simulink model "untitled"  (R2022b)
settings: Solver=VariableStepAuto  StartTime=0.0  StopTime=10.0  RelTol=1e-3
undefined symbols (not defined in the file): Ion, Lithium, Ts, Ts_Power
libraries: spsSeriesRLCBranchLib x7, spsMeanLib x5, spsFirstOrderFilterLib x4, spsStairGeneratorLib x4, spsDiodeLib x4, spsPWMGeneratorDCDCLib x3, spsBoostConverterLib x2, spsPVArrayLib x2, spsIGBTLib x2, spsPowerPositiveSequenceLib x1, spsRMSLib x1, spsBatteryLib x1
settings Model: Creator=刘明炜  LastModifiedBy=刘明炜

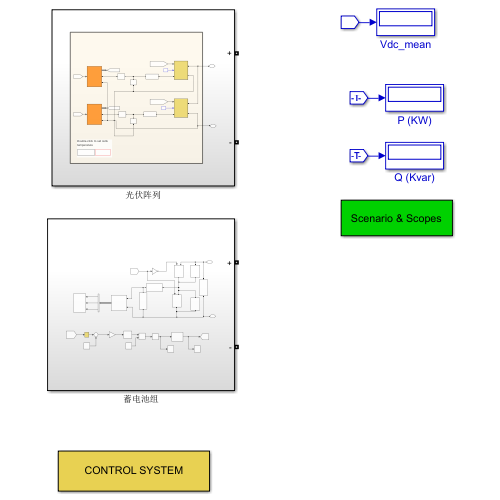
[thumbnail: Simulink's stored preview of the top-level diagram]
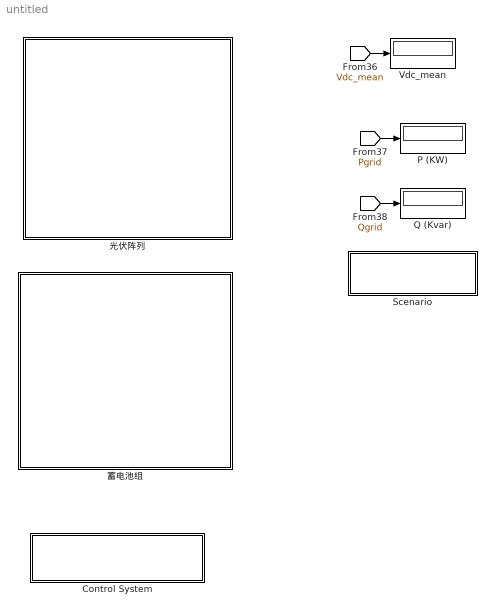
== system untitled ==
  Control System : Subsystem
      mask Display: disp('CONTROL SYSTEM')
  P (KW) : Display
      settings: Format=bank  Decimation=200
  Q (Kvar) : Display
      settings: Format=bank  Decimation=200
  Scenario : Subsystem
      mask Display: disp('Scenario & Scopes')
  Vdc_mean : Display
      settings: Decimation=200
  光伏阵列 : Subsystem
  蓄电池组 : Subsystem
  wires:
  [Pgrid] -> P (KW)/1
  [Vdc_mean] -> Vdc_mean/1
  [Qgrid] -> Q (Kvar)/1

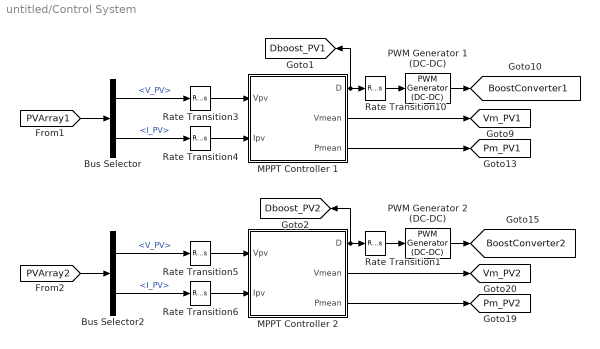
== system untitled/Control System ==
  Bus Selector : BusSelector  OutputSignals=V_PV,I_PV
  Bus Selector2 : BusSelector  OutputSignals=V_PV,I_PV
  MPPT Controller 1 : Subsystem  mask(MPPT Controller - Perturb and Observe algorithm (PandO)){Dinit=0.35, Dlimits=[0.8, 0.3], deltaD=60e-6, Fc=1000, Ts=Ts}
      mask prompts: Dinit "Duty cycle (D) initial value"; Dlimits "D limits [Upper, Lower]"; deltaD "Increment value for PandO algorithm"; Fc "Measurement filter cutoff frequency (Hz)"; Ts "Sample time (s)"
      mask init:
      | Dmax=Dlimits(1);
      | Dmin=Dlimits(2);
  MPPT Controller 2 : Subsystem  mask(MPPT Controller - Perturb and Observe algorithm (PandO)){Dinit=0.55, Dlimits=[0.8, 0.47], deltaD=60e-6, Fc=1000, Ts=Ts}
      mask prompts: Dinit "Duty cycle (D) initial value"; Dlimits "D limits [Upper, Lower]"; deltaD "Increment value for PandO algorithm"; Fc "Measurement filter cutoff frequency (Hz)"; Ts "Sample time (s)"
      mask init:
      | Dmax=Dlimits(1);
      | Dmin=Dlimits(2);
  PWM Generator 1 (DC-DC) : spsPWMGeneratorDCDCLib/PWM Generator (DC-DC)  Fsw=5000  Ts=Ts_Power
  PWM Generator 2 (DC-DC) : spsPWMGeneratorDCDCLib/PWM Generator (DC-DC)  Fsw=5000  Ts=Ts_Power
  Rate Transition1 : RateTransition  OutPortSampleTime=Ts_Power
  Rate Transition10 : RateTransition  OutPortSampleTime=Ts_Power
  Rate Transition{3..6} (4 alike) : RateTransition  OutPortSampleTime=Ts
  tag scope: BoostConverter1=global, BoostConverter2=global, Dboost_PV1=global, Dboost_PV2=global, Pm_PV1=global, Pm_PV2=global, Vm_PV1=global, Vm_PV2=global
  wires:
  MPPT Controller 2/2(Vmean) -> [Vm_PV2]
  Bus Selector2/1 -> Rate Transition5/1  "<V_PV>"
  Rate Transition3/1 -> MPPT Controller 1/1(Vpv)
  Rate Transition4/1 -> MPPT Controller 1/2(Ipv)
  Bus Selector/2 -> Rate Transition4/1  "<I_PV>"
  MPPT Controller 2/3(Pmean) -> [Pm_PV2]
  MPPT Controller 1/1(D) -> [Dboost_PV1], Rate Transition10/1
  Bus Selector/1 -> Rate Transition3/1  "<V_PV>"
  Bus Selector2/2 -> Rate Transition6/1  "<I_PV>"
  Rate Transition1/1 -> PWM Generator 2 (DC-DC)/1
  Rate Transition6/1 -> MPPT Controller 2/2(Ipv)
  MPPT Controller 1/3(Pmean) -> [Pm_PV1]
  MPPT Controller 1/2(Vmean) -> [Vm_PV1]
  Rate Transition10/1 -> PWM Generator 1 (DC-DC)/1
  MPPT Controller 2/1(D) -> [Dboost_PV2], Rate Transition1/1
  Rate Transition5/1 -> MPPT Controller 2/1(Vpv)
  PWM Generator 1 (DC-DC)/1 -> [BoostConverter1]
  PWM Generator 2 (DC-DC)/1 -> [BoostConverter2]
  [PVArray1] -> Bus Selector/1
  [PVArray2] -> Bus Selector2/1

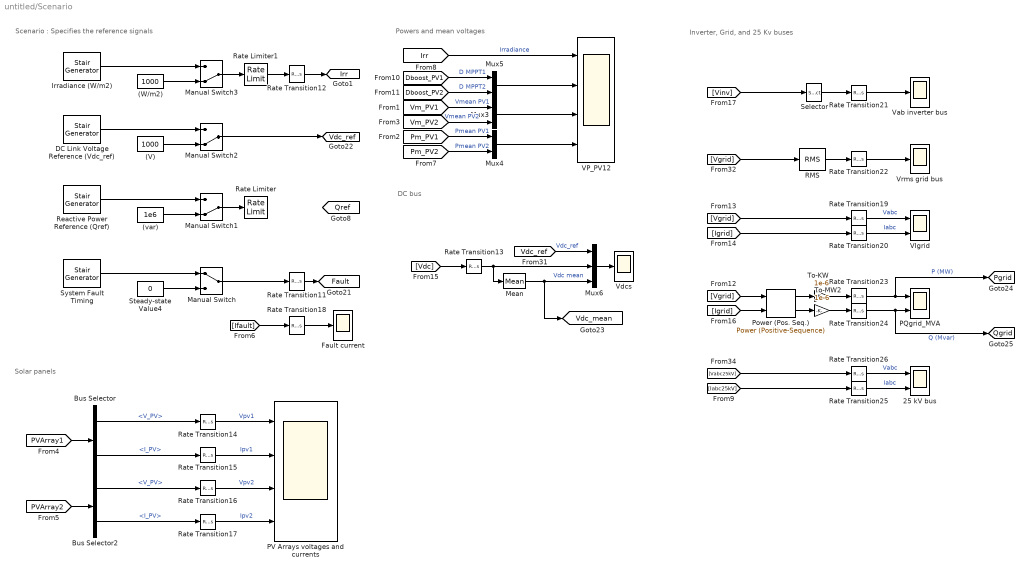
== system untitled/Scenario ==
  note: DC bus
  note: Powers and mean voltages
  note: Inverter, Grid, and 25 Kv buses
  note: Solar panels
  note: Scenario : Specifies the reference signals
  (V) : Constant  Value=1000
  (W/m2) : Constant  Value=1000
  (var) : Constant  Value=1e6
  25 kV bus : Scope  NumInputPorts=2
  Bus Selector : BusSelector  OutputSignals=V_PV,I_PV
  Bus Selector2 : BusSelector  OutputSignals=V_PV,I_PV
  DC Link Voltage Reference (Vdc_ref) : spsStairGeneratorLib/Stair Generator  t=[0, 0.2, 0.4]  e=[1000, 1050, 1000]  Ts=Ts
  Fault current : Scope
  Irradiance (W/m2) : spsStairGeneratorLib/Stair Generator  t=[0, 0.2, 0.4]  e=[1000, 250,1000]  Ts=Ts
  Manual Switch : ManualSwitch
  Manual Switch1 : ManualSwitch  CurrentSetting=0
  Manual Switch2 : ManualSwitch  CurrentSetting=0
  Manual Switch3 : ManualSwitch  CurrentSetting=0
  Mean : spsMeanLib/Mean  Freq=60  Vinit=1000  Ts=Ts
  Mux3 : Mux  Inputs=2
  Mux4 : Mux  Inputs=2
  Mux5 : Mux  Inputs=2
  Mux6 : Mux  Inputs=3
  PQgrid_MVA : Scope  NumInputPorts=2
  PV Arrays voltages and currents : Scope  NumInputPorts=4
  Power (Pos. Seq.) : spsPowerPositiveSequenceLib/Power (Positive-Sequence)  Freq=50  Vinit=[20570,-37]  Iinit=[70, -63]  Ts=Ts_Power
      settings: LibrarySourceBlock=|
      | sps_lib/Sensors and Measurements/Power
      | (Positive-Sequence)
  RMS : spsRMSLib/RMS  TrueRMS=off  Freq=50  RMSInit=25000  Ts=Ts_Power
  Rate Limiter : RateLimiter  RisingSlewLimit=1e6/(1/60)  FallingSlewLimit=-1e6/(1/60)  SampleTimeMode=inherited  InitialCondition=1e6
  Rate Limiter1 : RateLimiter  RisingSlewLimit=1000/(1/60)  FallingSlewLimit=-1000/(1/60)  SampleTimeMode=inherited  InitialCondition=1000
  Rate Transition11 : RateTransition  OutPortSampleTime=Ts_Power
  Rate Transition12 : RateTransition  OutPortSampleTime=Ts_Power
  Rate Transition{13..26} (14 alike) : RateTransition  OutPortSampleTime=Ts
  "Reactive Power Reference (Qref) " : spsStairGeneratorLib/Stair Generator  t=[0, 0.2, 0.4]  e=[1e6, -1e6, 1e6]  Ts=Ts
  Selector : Selector  InputPortWidth=3  IndexOptions=Index vector (dialog)  Indices=1  OutputSizes=1
  Steady-state Value4 : Constant  Value=0
  System Fault Timing : spsStairGeneratorLib/Stair Generator  t=[0, 0.25, 0.45]  e=[0, 1, 0]  Ts=Ts
  To-KW : Gain  Gain=1e-6
  To-MW2 : Gain  Gain=1e-6
  VIgrid : Scope  NumInputPorts=2
  VP_PV12 : Scope  NumInputPorts=4
  Vab inverter bus : Scope
  Vdcs : Scope
  Vrms grid bus : Scope
  tag scope: Fault=global, Irr=global, Pgrid=global, Qgrid=global, Qref=global, Vdc_mean=global, Vdc_ref=global
  wires:
  (W/m2)/1 -> Manual Switch3/2
  (V)/1 -> Manual Switch2/2
  Steady-state Value4/1 -> Manual Switch/2
  DC Link Voltage Reference (Vdc_ref)/1 -> Manual Switch2/1
  System Fault Timing/1 -> Manual Switch/1
  Manual Switch/1 -> Rate Transition11/1
  Rate Limiter1/1 -> Rate Transition12/1
  (var)/1 -> Manual Switch1/2
  "Reactive Power Reference (Qref) "/1 -> Manual Switch1/1
  Manual Switch1/1 -> Rate Limiter/1
  Manual Switch2/1 -> [Vdc_ref]
  Irradiance (W/m2)/1 -> Manual Switch3/1
  Manual Switch3/1 -> Rate Limiter1/1
  Rate Transition12/1 -> [Irr]
  Bus Selector2/1 -> Rate Transition16/1  "<V_PV>"
  Bus Selector/2 -> Rate Transition15/1  "<I_PV>"
  Bus Selector/1 -> Rate Transition14/1  "<V_PV>"
  Rate Transition19/1 -> VIgrid/1  "Vabc"
  [Pm_PV1] -> Mux4/1  "Pmean PV1"
  Rate Transition17/1 -> PV Arrays voltages and currents/4  "Ipv2"
  RMS/1 -> Rate Transition22/1
  [Pm_PV2] -> Mux4/2  "Pmean PV2"
  [Irr] -> VP_PV12/1  "Irradiance"
  Rate Transition22/1 -> Vrms grid bus/1
  Rate Transition16/1 -> PV Arrays voltages and currents/3  "Vpv2"
  Rate Transition26/1 -> 25 kV bus/1  "Vabc"
  Mux3/1 -> VP_PV12/3
  [Vgrid] -> RMS/1
  [Vgrid] -> Power (Pos. Seq.)/1
  Rate Transition23/1 -> [Pgrid], PQgrid_MVA/1  "P (MW)"
  [PVArray1] -> Bus Selector/1
  Rate Transition20/1 -> VIgrid/2  "Iabc"
  Mux6/1 -> Vdcs/1
  Mux4/1 -> VP_PV12/4
  Rate Transition15/1 -> PV Arrays voltages and currents/2  "Ipv1"
  Mux5/1 -> VP_PV12/2
  Power (Pos. Seq.)/2 -> To-MW2/1
  [Igrid] -> Rate Transition20/1
  Rate Transition18/1 -> Fault current/1
  [Vabc25kV] -> Rate Transition26/1
  Rate Transition25/1 -> 25 kV bus/2  "Iabc"
  [Vm_PV2] -> Mux3/2  "Vmean PV2"
  Rate Transition14/1 -> PV Arrays voltages and currents/1  "Vpv1"
  [Vgrid] -> Rate Transition19/1
  Rate Transition13/1 -> Mean/1, Mux6/2
  Power (Pos. Seq.)/1 -> To-KW/1
  [Dboost_PV1] -> Mux5/1  "D MPPT1"
  [Vinv] -> Selector/1
  Mean/1 -> Mux6/3, [Vdc_mean]  "Vdc mean"
  Rate Transition11/1 -> [Fault]
  [Dboost_PV2] -> Mux5/2  "D MPPT2"
  [Vm_PV1] -> Mux3/1  "Vmean PV1"
  [Vdc_ref] -> Mux6/1  "Vdc_ref"
  [Igrid] -> Power (Pos. Seq.)/2
  Bus Selector2/2 -> Rate Transition17/1  "<I_PV>"
  [Iabc25kV] -> Rate Transition25/1
  Rate Transition24/1 -> [Qgrid], PQgrid_MVA/2  "Q (Mvar)"
  [Vdc] -> Rate Transition13/1
  [PVArray2] -> Bus Selector2/1
  [Ifault] -> Rate Transition18/1
  Selector/1 -> Rate Transition21/1
  Rate Transition21/1 -> Vab inverter bus/1
  To-MW2/1 -> Rate Transition24/1
  To-KW/1 -> Rate Transition23/1

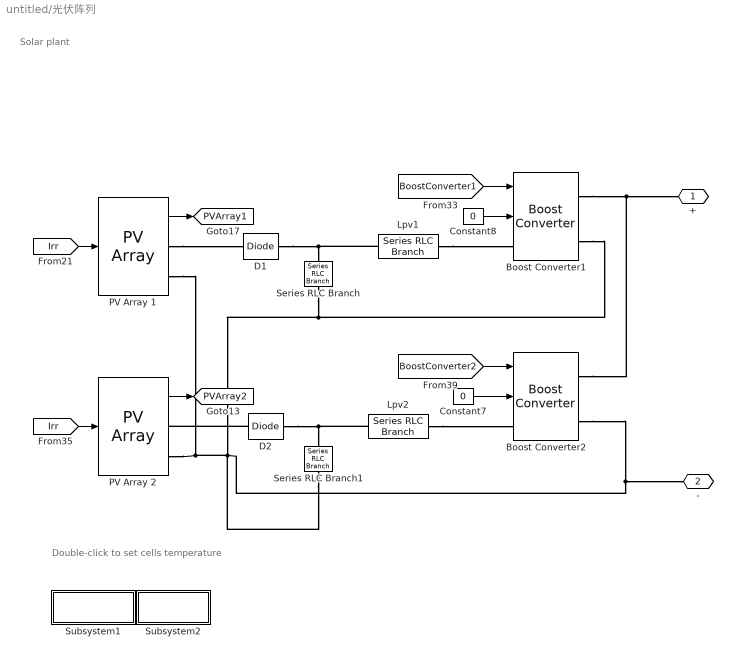
== system untitled/光伏阵列 ==
  note: Solar plant
  note: Double-click to set cells temperature
  Boost Converter1 : spsBoostConverterLib/Boost Converter  ModelType=Switching devices  Ron=1e-4  Rs=1e6  Cs=inf  Vforward=[0,0]  Ron_Diode=1e-4  Rs_Diode=1e6  Cs_Diode=inf  Vf_Diode=0  Rs_CurrentSource=inf  Ron_ACsource=1e-3
      settings: LibrarySourceBlock=sps_lib/Power Electronics/Boost Converter
  Boost Converter2 : spsBoostConverterLib/Boost Converter  ModelType=Switching devices  Ron=1e-4  Rs=1e6  Cs=inf  Vforward=[0,0]  Ron_Diode=1e-4  Rs_Diode=1e6  Cs_Diode=inf  Vf_Diode=0  Rs_CurrentSource=inf  Ron_ACsource=1e-3
      settings: LibrarySourceBlock=sps_lib/Power Electronics/Boost Converter
  Constant7 : Constant  Value=0  SampleTime=Ts
  Constant8 : Constant  Value=0  SampleTime=Ts
  D1 : spsDiodeLib/Diode  Ron=1e-4  Lon=0  Vf=0  IC=0  UseSnubber=0  Rs=1e6  Cs=inf  Measurements=off
  D2 : spsDiodeLib/Diode  Ron=1e-4  Lon=0  Vf=0  IC=0  UseSnubber=0  Rs=1e6  Cs=inf  Measurements=off
  Lpv1 : spsSeriesRLCBranchLib/Series RLC Branch  LConnTagsString=__new0  RConnTagsString=__new0  BranchType=RL  Resistance=1e-3  Inductance=1e-3  SetiL0=off  InitialCurrent=0  Capacitance=120e-3  Setx0=off  InitialVoltage=0  Measurements=None
  Lpv2 : spsSeriesRLCBranchLib/Series RLC Branch  LConnTagsString=__new0  RConnTagsString=__new0  BranchType=RL  Resistance=1e-3  Inductance=1e-3  SetiL0=off  InitialCurrent=0  Capacitance=120e-3  Setx0=off  InitialVoltage=0  Measurements=None
  PV Array 1 : spsPVArrayLib/PV Array  Npar=282  Nser=15  PlotType=array @ 1000 W/m2 & specified temperatures  S_vec=[ 1000 250]  Temp_C_vec="[ 45 25  ]"  ModuleName=User-defined  PlotWhenSelected=off  Pm=355.012  Ncell=83  Voc=51.9  Isc=8.68  Vm=43.4  Im=8.18  beta_Voc_pc=-0.304  alpha_Isc_pc=0.017  beta_Voc=-0.15778  alpha_Isc=0.0014756  IL=8.6865  I0=3.3093e-11  nI=0.92618  Rsh=389.4331  Rs=0.29289  RobustModel=on  RobustCellTemperature=25  BAL=on  Tc=1e-6  Tfilter=5e-5
      settings: AttributesFormatString=(%<RobustCellTemperature> deg. C)
  PV Array 2 : spsPVArrayLib/PV Array  Npar=122  Nser=14  PlotType=array @ 1000 W/m2 & specified temperatures  S_vec=[ 1000 250]  Temp_C_vec="[ 45 25  ]"  ModuleName=User-defined  PlotWhenSelected=off  Pm=293.664  Ncell=60  Voc=39.5  Isc=9.60  Vm=32.2  Im=9.12  beta_Voc_pc=-0.300  alpha_Isc_pc=0.03  beta_Voc=-0.1185  alpha_Isc=0.00288  IL=9.6627  I0=3.1923e-11  nI=0.96973  Rsh=336.4947  Rs=0.3029  RobustModel=on  RobustCellTemperature=25  BAL=on  Tc=1e-6  Tfilter=5e-5
      settings: AttributesFormatString=(%<RobustCellTemperature> deg. C)
  Series RLC Branch : spsSeriesRLCBranchLib/Series RLC Branch  LConnTagsString=__new0  RConnTagsString=__new0  BranchType=C  Resistance=1  Inductance=1e-3  SetiL0=off  InitialCurrent=0  Capacitance=200e-6  Setx0=on  InitialVoltage=650  Measurements=None
  Series RLC Branch1 : spsSeriesRLCBranchLib/Series RLC Branch  LConnTagsString=__new0  RConnTagsString=__new0  BranchType=C  Resistance=1  Inductance=1e-3  SetiL0=off  InitialCurrent=0  Capacitance=200e-6  Setx0=on  InitialVoltage=450  Measurements=None
  Subsystem1 : Subsystem
      settings: OpenFcn=|
      | SystemName1=gcs;
      | BlockName1=[SystemName1, '/', 'PV Array 1'];
      | set_param(BlockName1,'RobustCellTemperature','25');
      | set_param(BlockName1,'ForegroundColor','black');
      | BlockName2=[SystemName1, '/', 'PV Array 2'];
      | set_param(BlockName2,'RobustCellTemperature','25');
      | set_param(BlockName2,'ForegroundColor','black');
      mask Display: disp('25 deg. C')
  Subsystem2 : Subsystem
      settings: OpenFcn=|
      | SystemName1=gcs;
      | BlockName1=[SystemName1, '/', 'PV Array 1'];
      | set_param(BlockName1,'RobustCellTemperature','45');
      | set_param(BlockName1,'ForegroundColor','red');
      | BlockName2=[SystemName1, '/', 'PV Array 2'];
      | set_param(BlockName2,'RobustCellTemperature','45');
      | set_param(BlockName2,'ForegroundColor','red');
      mask Display: disp('45 deg. C')
  + : PMIOPort  Side=Right
  - : PMIOPort  Port=2  Side=Right
  tag scope: PVArray1=global, PVArray2=global
  wires:
  [BoostConverter2] -> Boost Converter2/1
  [BoostConverter1] -> Boost Converter1/1
  PV Array 1/1 -> [PVArray1]
  PV Array 2/1 -> [PVArray2]
  [Irr] -> PV Array 2/1
  Constant8/1 -> Boost Converter1/2
  [Irr] -> PV Array 1/1
  Constant7/1 -> Boost Converter2/2
  connections:
  D1/RConn1 -- Series RLC Branch/LConn1 -- Lpv1/RConn1
  Boost Converter1/RConn1 -- Boost Converter2/RConn1 -- +/RConn1
  Series RLC Branch1/RConn1 -- PV Array 2/RConn2 -- PV Array 1/RConn2 -- Series RLC Branch/RConn1 -- Boost Converter1/RConn2 -- Boost Converter2/RConn2 -- -/RConn1
  D2/RConn1 -- Series RLC Branch1/LConn1 -- Lpv2/RConn1
  Lpv2/LConn1 -- Boost Converter2/LConn1
  PV Array 1/RConn1 -- D1/LConn1
  Lpv1/LConn1 -- Boost Converter1/LConn1
  D2/LConn1 -- PV Array 2/RConn1

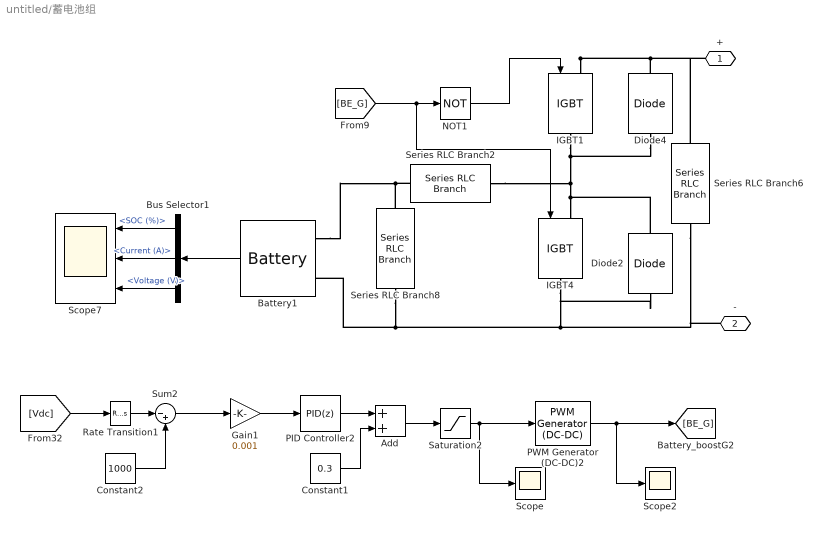
== system untitled/蓄电池组 ==
  Add : Sum
  Battery1 : spsBatteryLib/Battery  BatType=Lithium-Ion  ShowTempParam=off  ThermalPreset=no  ShowAgeParam=off  NomV=300  NomQ=100  SOC=100  Batt_Tr=0.1  PresetModel=on  MaxQ=100  MinV=225  FullV=349.1961  Dis_rate=43.4783  R=0.03  Normal_OP=90.4348  expZone="[324.1158      4.913043]"  current=[6.5 13 32.5]  Units=Time  Tci=20  NomT=20  T2=-30  MaxQ2=4.8  FullV2=7.1  Normal_OP2=5.655  expZone2="[6.58           1]"  Rca=0.6  ti=2000  Dp=0  Neq0=0  Tsim=1e6  Ta1=25  Qeol=5.4*0.9  Reol=0.013333*1.2  Char_age=[2.3478, 3]  Dis_age=[2.3478, 10]  N1=1500  N2=10500  N3=1000  N4=1400  Ta2=45  N5=950
  Bus Selector1 : BusSelector  OutputSignals=SOC (%),Current (A),Voltage (V)
  Constant1 : Constant  Value=0.3
  Constant2 : Constant  Value=1000
  Diode2 : spsDiodeLib/Diode  Ron=0.001  Lon=0  Vf=0.8  IC=0  UseSnubber=off  Rs=500  Cs=250e-9  Measurements=off
  Diode4 : spsDiodeLib/Diode  Ron=0.001  Lon=0  Vf=0.8  IC=0  UseSnubber=off  Rs=500  Cs=250e-9  Measurements=off
  Gain1 : Gain  Gain=0.001
  IGBT1 : spsIGBTLib/IGBT  Ron=0.001  Lon=0  Vf=1  Tf=1e-6  Tt=2e-6  IC=0  Rs=1e5  Cs=inf  Measurements=off
  IGBT4 : spsIGBTLib/IGBT  Ron=0.001  Lon=0  Vf=1  Tf=1e-6  Tt=2e-6  IC=0  Rs=1e5  Cs=inf  Measurements=off
  NOT1 : Logic  Operator=NOT  IconShape=distinctive  AllPortsSameDT=off  OutDataTypeStr=boolean
  PID Controller2 : slpidlib/PID Controller  Controller=PID  Form=Parallel  TimeDomain=Discrete-time  UseExternalTs=off  SampleTime=-1  IntegratorMethod=Forward Euler  FilterMethod=Forward Euler  ControllerParametersSource=internal  P=2  I=4  UseKiTs=off  D=0.008  N=100  UseFilter=on  TunerSelectOption=Transfer Function Based (PID Tuner App)  InitialConditionSource=internal  InitialConditionForIntegrator=0  InitialConditionForFilter=0  DifferentiatorICPrevScaledInput=0  ExternalReset=none  TrackingMode=off  Kt=1  LimitOutput=off  SatLimitsSource=internal  UpperSaturationLimit=0.1  LowerSaturationLimit=-0.1  LinearizeAsGain=off  AntiWindupMode=clamping  Kb=1  LimitIntegrator=off  UpperIntegratorSaturationLimit=5  LowerIntegratorSaturationLimit=-5  POutMin=[]  POutMax=[]  IOutMin=[]  IOutMax=[]  DOutMin=[]  DOutMax=[]  NOutMin=[]  NOutMax=[]  SumOutMin=[]  SumOutMax=[]  SaturationOutMin=[]  SaturationOutMax=[]  PParamMin=[]  PParamMax=[]  IParamMin=[]  IParamMax=[]  DParamMin=[]  DParamMax=[]  NParamMin=[]  NParamMax=[]  KbParamMin=[]  KbParamMax=[]  KtParamMin=[]  KtParamMax=[]  KbOutMin=[]  KbOutMax=[]  KtOutMin=[]  KtOutMax=[]  IntegratorOutMin=[]  IntegratorOutMax=[]  FilterOutMin=[]  FilterOutMax=[]  SumI1OutMin=[]  SumI1OutMax=[]  SumI2OutMin=[]  SumI2OutMax=[]  SumI3OutMin=[]  SumI3OutMax=[]  SumI4OutMin=[]  SumI4OutMax=[]  SumDOutMin=[]  SumDOutMax=[]  DifferentiatorOutMin=[]  DifferentiatorOutMax=[]  FilterDiffOutCoefMin=[]  FilterDiffOutCoefMax=[]  ReciprocalOutMin=[]  ReciprocalOutMax=[]  SumDenOutMin=[]  SumDenOutMax=[]  SumNumOutMin=[]  SumNumOutMax=[]  DivideOutMin=[]  DivideOutMax=[]  UdiffTsProdOutMin=[]  UdiffTsProdOutMax=[]  NTsProdOutMin=[]  NTsProdOutMax=[]  UintegralTsProdOutMin=[]  UintegralTsProdOutMax=[]  UngainTsProdOutMin=[]  UngainTsProdOutMax=[]  ClampingZeroOutDataTypeStr=Inherit: Inherit via back propagation  ClampingZeroOutMin=[]  ClampingZeroOutMax=[]  FilterDenConstantOutDataTypeStr=Inherit: Inherit via back propagation  FilterDenConstantOutMin=[]  FilterDenConstantOutMax=[]  PCopyOutDataTypeStr=Inherit: Inherit via back propagation  PCopyOutMin=[]  PCopyOutMax=[]  NCopyOutDataTypeStr=Inherit: Inherit via back propagation  NCopyOutMin=[]  NCopyOutMax=[]  IntegratorContinuousStateAttributes=''  IntegratorStateMustResolveToSignalObject=off  IntegratorRTWStateStorageClass=Auto  FilterContinuousStateAttributes=''  FilterStateMustResolveToSignalObject=off  FilterRTWStateStorageClass=Auto  ParallelPVariant=InternalParameters  IdealPVariant=Disabled  IVariant=InternalParameters  DVariant=InternalParameters  IntegratorVariant=Discrete  SatVariant=Disabled  AWVariant=Passthrough  PCopyVariant=Disabled  TRVariant=Disabled  FdbkBlocksVariant=Forward  IdealPFdbkVariant=Disabled  SatFdbkVariant=Disabled  DerivativeFilterVariant=ForwardEulerFilter  NVariant=InternalParameters  NCopyVariant=Disabled  FilterICVariant=InternalICsFilter  IntegratorICVariant=InternalICs  ExternalResetVariant=Disabled  TRSumVariant=Passthrough  SumFdbkVariant=Disabled  SumVariant=Sum_PID  TsampFilterVariant=InternalTs  TsampNgainVariant=Passthrough  TsampIntegralVariant=Passthrough  ExternalSaturationOutDataTypeStr=Inherit: Same as second input
  PWM Generator (DC-DC)2 : spsPWMGeneratorDCDCLib/PWM Generator (DC-DC)  Fsw=10000  Ts=0
  Rate Transition1 : RateTransition  OutPortSampleTime=50e-6
  Saturation2 : Saturate  UpperLimit=0.9  LowerLimit=0.01
  Scope : Scope
  Scope2 : Scope
  Scope7 : Scope  NumInputPorts=3
  Series RLC Branch2 : spsSeriesRLCBranchLib/Series RLC Branch  LConnTagsString=__new0  RConnTagsString=__new0  BranchType=L  Resistance=1  Inductance=0.002  SetiL0=off  InitialCurrent=0  Capacitance=1e-6  Setx0=off  InitialVoltage=0  Measurements=None
  Series RLC Branch6 : spsSeriesRLCBranchLib/Series RLC Branch  LConnTagsString=__new0  RConnTagsString=__new0  BranchType=C  Resistance=1  Inductance=1e-3  SetiL0=off  InitialCurrent=0  Capacitance=470e-4  Setx0=off  InitialVoltage=0  Measurements=None
  Series RLC Branch8 : spsSeriesRLCBranchLib/Series RLC Branch  LConnTagsString=__new0  RConnTagsString=__new0  BranchType=C  Resistance=1  Inductance=1e-3  SetiL0=off  InitialCurrent=0  Capacitance=470e-6  Setx0=off  InitialVoltage=0  Measurements=None
  Sum2 : Sum  Inputs=|-+
  + : PMIOPort  Side=Right
  - : PMIOPort  Port=2  Side=Right
  wires:
  Saturation2/1 -> Scope/1, PWM Generator (DC-DC)2/1
  Bus Selector1/2 -> Scope7/2  "<Current (A)>"
  Rate Transition1/1 -> Sum2/1
  Constant2/1 -> Sum2/2
  Add/1 -> Saturation2/1
  Constant1/1 -> Add/2
  [BE_G] -> IGBT4/1, NOT1/1
  Sum2/1 -> Gain1/1
  PID Controller2/1 -> Add/1
  Bus Selector1/1 -> Scope7/1  "<SOC (%)>"
  [Vdc] -> Rate Transition1/1
  Gain1/1 -> PID Controller2/1
  NOT1/1 -> IGBT1/1
  Battery1/1 -> Bus Selector1/1
  PWM Generator (DC-DC)2/1 -> Scope2/1, [BE_G]
  Bus Selector1/3 -> Scope7/3  "<Voltage (V)>"
  connections:
  IGBT1/RConn1 -- Diode4/LConn1 -- Series RLC Branch2/RConn1 -- Diode2/RConn1 -- IGBT4/LConn1
  Series RLC Branch2/LConn1 -- Series RLC Branch8/LConn1 -- Battery1/LConn1
  Series RLC Branch8/RConn1 -- Battery1/LConn2 -- Diode2/LConn1 -- IGBT4/RConn1 -- -/RConn1 -- Series RLC Branch6/RConn1
  IGBT1/LConn1 -- Diode4/RConn1 -- +/RConn1 -- Series RLC Branch6/LConn1

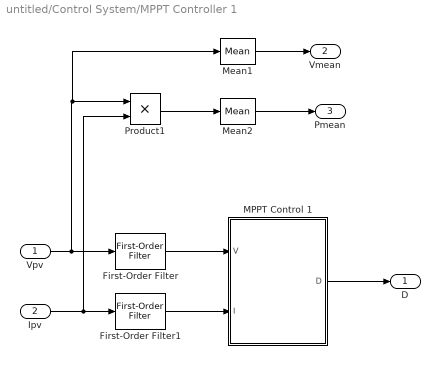
== system untitled/Control System/MPPT Controller 1 ==
  Vpv : Inport
  Ipv : Inport  Port=2
  First-Order Filter : spsFirstOrderFilterLib/First-Order Filter  FilterType=Lowpass  Tc=1/Fc  Ts=Ts  Initialize=off  Vac_Init=[0, 0, 60]  Vdc_Init=0  PlotResponse=off  FreqRange="[0,  200,  1]"
  First-Order Filter1 : spsFirstOrderFilterLib/First-Order Filter  FilterType=Lowpass  Tc=1/Fc  Ts=Ts  Initialize=off  Vac_Init=[0, 0, 60]  Vdc_Init=0  PlotResponse=off  FreqRange="[0,  200,  1]"
  "MPPT Control 1 " : MATLAB Function  TreatAsAtomicUnit=on
  Mean1 : spsMeanLib/Mean  Freq=60  Vinit=650  Ts=Ts
  Mean2 : spsMeanLib/Mean  Freq=60  Vinit=1500e3  Ts=Ts
  Product1 : Product
  D : Outport  VectorParamsAs1DForOutWhenUnconnected=off
  Vmean : Outport  Port=2  VectorParamsAs1DForOutWhenUnconnected=off
  Pmean : Outport  Port=3  VectorParamsAs1DForOutWhenUnconnected=off
  wires:
  First-Order Filter1/1 -> "MPPT Control 1 "/2(I)
  First-Order Filter/1 -> "MPPT Control 1 "/1(V)
  Ipv/1 -> Product1/2, First-Order Filter1/1
  Vpv/1 -> Mean1/1, Product1/1, First-Order Filter/1
  "MPPT Control 1 "/1(D) -> D/1
  Product1/1 -> Mean2/1
  Mean1/1 -> Vmean/1
  Mean2/1 -> Pmean/1

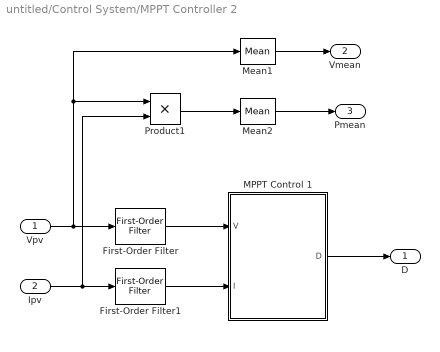
== system untitled/Control System/MPPT Controller 2 ==
  Vpv : Inport
  Ipv : Inport  Port=2
  First-Order Filter : spsFirstOrderFilterLib/First-Order Filter  FilterType=Lowpass  Tc=1/Fc  Ts=Ts  Initialize=off  Vac_Init=[0, 0, 60]  Vdc_Init=0  PlotResponse=off  FreqRange="[0,  200,  1]"
  First-Order Filter1 : spsFirstOrderFilterLib/First-Order Filter  FilterType=Lowpass  Tc=1/Fc  Ts=Ts  Initialize=off  Vac_Init=[0, 0, 60]  Vdc_Init=0  PlotResponse=off  FreqRange="[0,  200,  1]"
  "MPPT Control 1 " : MATLAB Function  TreatAsAtomicUnit=on
  Mean1 : spsMeanLib/Mean  Freq=60  Vinit=420  Ts=Ts
  Mean2 : spsMeanLib/Mean  Freq=60  Vinit=500e3  Ts=Ts
  Product1 : Product
  D : Outport  VectorParamsAs1DForOutWhenUnconnected=off
  Vmean : Outport  Port=2  VectorParamsAs1DForOutWhenUnconnected=off
  Pmean : Outport  Port=3  VectorParamsAs1DForOutWhenUnconnected=off
  wires:
  "MPPT Control 1 "/1(D) -> D/1
  Ipv/1 -> Product1/2, First-Order Filter1/1
  First-Order Filter/1 -> "MPPT Control 1 "/1(V)
  First-Order Filter1/1 -> "MPPT Control 1 "/2(I)
  Mean1/1 -> Vmean/1
  Product1/1 -> Mean2/1
  Mean2/1 -> Pmean/1
  Vpv/1 -> Product1/1, Mean1/1, First-Order Filter/1

== system untitled/光伏阵列/Subsystem1 ==

== system untitled/光伏阵列/Subsystem2 ==

== matlab function untitled/Control System/MPPT Controller 2/MPPT Control 1  ==
  settings: updateMethod=DISCRETE  sampleTime=Ts
  data: V input =V; I input; D output; Dmax parameter; Dmin parameter; deltaD parameter; Dinit parameter
function D  = PandO(V, I, Dmax, Dmin, deltaD, Dinit)

% MPPT controller based on the Perturb & Observe algorithm.

% D output = Duty cycle of the boost converter (value between 0 and 1)
% V input = PV array terminal voltage (V)
% I input = PV array current (A)
% D = 1 - Vinput/Voutput (increasing D decrease Vin)

persistent Vold Pold Dold;
%
if isempty(Vold)
    Vold=0;
    Pold=0;
    Dold=Dinit;
end
P= V*I;
dV= V - Vold;
dP= P - Pold;
%
% if dP ~= 0
    if dP < 0
        if dV < 0
            D = Dold - deltaD;
        else
            D = Dold + deltaD;
        end
    else
        if dV < 0
            D = Dold + deltaD;
        else
            D = Dold - deltaD;
        end    
    end
% else
%     D=Dold;
% end
%
if D >= Dmax || D<= Dmin
    D=Dold;
end
%
Dold=D;
Vold=V;
Pold=P;

== matlab function untitled/Control System/MPPT Controller 1/MPPT Control 1  ==
  settings: updateMethod=DISCRETE  sampleTime=Ts
  data: V input =V; I input; D output; Dmax parameter; Dmin parameter; deltaD parameter; Dinit parameter
function D  = PandO(V, I, Dmax, Dmin, deltaD, Dinit)

% MPPT controller based on the Perturb & Observe algorithm.

% D output = Duty cycle of the boost converter (value between 0 and 1)
% V input = PV array terminal voltage (V)
% I input = PV array current (A)
% D = 1 - Vinput/Voutput (increasing D decrease Vin)

persistent Vold Pold Dold;
%
if isempty(Vold)
    Vold=0;
    Pold=0;
    Dold=Dinit;
end
P= V*I;
dV= V - Vold;
dP= P - Pold;
%
% if dP ~= 0
    if dP < 0
        if dV < 0
            D = Dold - deltaD;
        else
            D = Dold + deltaD;
        end
    else
        if dV < 0
            D = Dold + deltaD;
        else
            D = Dold - deltaD;
        end    
    end
% else
%     D=Dold;
% end
%
if D >= Dmax || D<= Dmin
    D=Dold;
end
%
Dold=D;
Vold=V;
Pold=P;
